simulink model "DDR"  (R2021a)
settings: Solver=VariableStepAuto  StartTime=0.0  StopTime=10.0  RelTol=1e-3
values from neighbouring files (symbols this model uses):
  sampleTime = 0.01    [Discrete.m]
libraries: mobileRoboticsLib x4
settings Model: Creator=dabc  LastModifiedBy=dabc

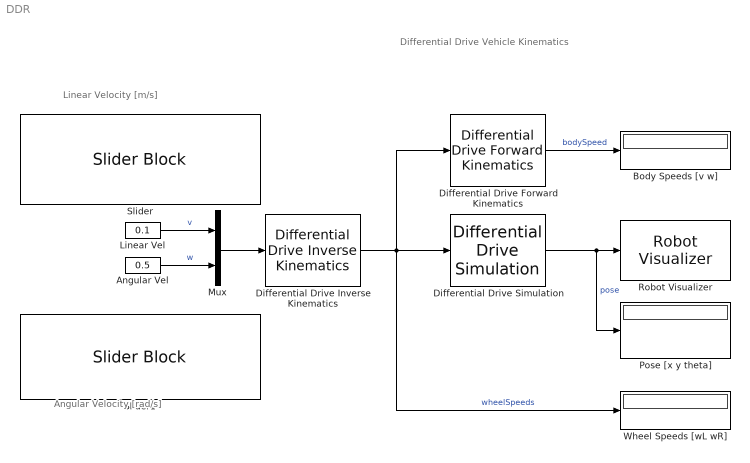
== system DDR ==
  note: Angular Velocity [rad/s]
  note: Differential Drive Vehicle Kinematics
  note: Linear Velocity [m/s]
  Angular Vel : Constant  Value=0.5
  Body Speeds [v w] : Display
  Differential Drive Forward Kinematics : mobileRoboticsLib/Kinematic Models/Differential Drive/Differential Drive Forward Kinematics  wheelRadius=R  wheelBase=L
      settings: SourceProductName=Mobile Robotics Simulation Library
  Differential Drive Inverse Kinematics : mobileRoboticsLib/Kinematic Models/Differential Drive/Differential Drive Inverse Kinematics  wheelRadius=R  wheelBase=L
      settings: SourceProductName=Mobile Robotics Simulation Library
  Differential Drive Simulation : mobileRoboticsLib/Kinematic Models/Differential Drive/Differential Drive Simulation  wheelRadius=R  wheelBase=L  initX=0  initY=0  initAngle=0  Ts=sampleTime
      settings: SourceProductName=Mobile Robotics Simulation Library
  Linear Vel : Constant  Value=0.1
  Mux : Mux  Inputs=2
  Pose [x y theta] : Display
  Robot Visualizer : mobileRoboticsLib/Environments/Robot Visualizer  Priority=99  robotRadius=0  showTrajectory=on  hasWaypoints=off  hasLidar=off  sensorOffset=[ 0 0 ]  scanAngles=scanAngles  hasObjDetector=off  objDetectorOffset=[ 0, 0 ]  objDetectorAngle=0  objDetectorFOV=pi/4  objDetectorMaxRange=5  objectColors=[ 1, 0, 0; 0, 1, 0; 0, 0, 1 ]  objectMarkers=s
      settings: SourceProductName=Mobile Robotics Simulation Library
  Slider : SliderBlock  ScaleMin=-1  ScaleMax=1  TickInterval=0.25
  Slider1 : SliderBlock  ScaleMin=-1.5  ScaleMax=1.5
  Wheel Speeds [wL wR] : Display
  wires:
  Differential Drive Inverse Kinematics/1 -> Differential Drive Simulation/1, Differential Drive Forward Kinematics/1, Wheel Speeds [wL wR]/1  "wheelSpeeds"
  Mux/1 -> Differential Drive Inverse Kinematics/1
  Differential Drive Simulation/1 -> Pose [x y theta]/1, Robot Visualizer/1  "pose"
  Angular Vel/1 -> Mux/2  "w"
  Linear Vel/1 -> Mux/1  "v"
  Differential Drive Forward Kinematics/1 -> Body Speeds [v w]/1  "bodySpeed"
